simulink model "rtwdemo_shrlib"  (Simulink 7.6)
settings: Solver=FixedStepDiscrete  SolverMode=SingleTasking  StartTime=0.0  StopTime=inf  FixedStep=1  RelTol=1e-3
PostLoadFcn:
  | INC=uint8(1);LIMIT=uint8(4);RESET=uint8(0);K=int32(3);
  | addpath(fullfile((matlabroot), 'toolbox', 'rtw', 'rtwdemos', 'shrlib_demo'));
libraries: rtwdemowidgets x1
Description:
  | Interfacing to Host Simulators Using Shared Libraries
settings Model: Creator=The MathWorks Inc.  ParamWorkspaceSource=ReferencedWorkspace  CovMetricSettings=d  ExtModeTrigMode=oneshot  ExtModeArmWhenConnect=off  ExtModeAutoUpdateStatusClock=off
settings MATStruct: SampleTime=1  Offset=0  Priority=[41.0]
settings DataIOCC: LimitDataPoints=off  SignalLogging=off  SignalLoggingName=sigsOut
settings OptimizationCC: InlineParams=on  InlineInvariantSignals=on  PassReuseOutputArgsAs=Individual arguments  StateBitsets=on  DataBitsets=on  UseTempVars=on  ZeroExternalMemoryAtStartup=off  ZeroInternalMemoryAtStartup=off  NoFixptDivByZeroProtection=on  EfficientFloat2IntCast=on  EfficientMapNaN2IntZero=off  OptimizeModelRefInitCode=on  LifeSpan=1  BufferReusableBoundary=off
settings DebuggingCC: CheckExecutionContextPreStartOutputMsg=on  CheckExecutionContextRuntimeOutputMsg=on  SolverPrmCheckMsg=none  IntegerOverflowMsg=none  StrictBusMsg=ErrorOnBusTreatedAsVector
settings HardwareCC: ProdIntDivRoundTo=Zero  ProdEndianess=LittleEndian  ProdHWDeviceType=Generic->32-bit Embedded Processor  TargetHWDeviceType=Generic->32-bit Embedded Processor
settings ModelReferenceCC: UpdateModelReferenceTargets=IfOutOfDate
settings RTWCC: SystemTargetFile=ert_shrlib.tlc  TLCOptions=-p0 -aWarnNonSaturatedBlocks=0  TemplateMakefile=ert_default_tmf  Description=Real-Time Workshop Embedded Coder (host-based shared library target)  RTWVerbose=off  ProcessScript=ert_shrlib_make_rtw_hook
settings CodeAppCC: ForceParamTrailComments=on  IgnoreCustomStorageClasses=off  IgnoreTestpoints=on
settings STFCustomTargetCC: TargetFcnLib=ansi_tfl_tmw.mat  ParMdlRefBuildCompliant=on  CompOptLevelCompliant=on  CombineOutputUpdateFcns=on  ERTCustomFileBanners=on  SupportNonFinite=off  SupportContinuousTime=off  SupportNonInlinedSFcns=off  ModelStepFunctionPrototypeControlCompliant=on  CPPClassGenCompliant=on  SystemTargetFile=ert_shrlib.tlc
settings ERTTargetCC: TargetFcnLib=ansi_tfl_tmw.mat  MultiwordLength=2048  ERTFirstTimeCompliant=off  SupportNonFinite=off  ExtModeMexFile=noextcomm  InlinedParameterPlacement=NonHierarchical  ERTCustomFileTemplate=example_file_process.tlc  ERTFilePackagingFormat=CompactWithDataFile  ConvertIfToSwitch=off

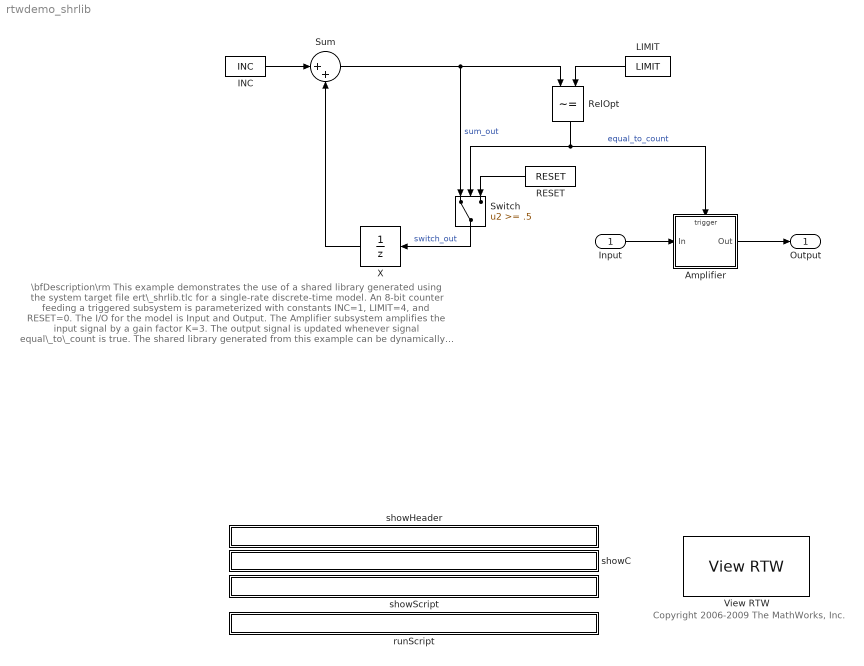
== system rtwdemo_shrlib ==
  note: \bfDescription\rm
      | This example demonstrates the use of a shared library generated using the system target file
      | ert\_shrlib.tlc for a single-rate discrete-time model. An 8-bit counter feeding a triggered
      | subsystem is parameterized with constants INC=1, LIMIT=4, and RESET=0.  The I/O for the model
      | is Input and Output. The Amplifier subsystem amplifies the input signal by a gain factor K=3. The
      | output signal is updated whenever signal equal\_to\_count is true. The shared library generated
      | from this example can be dynamically loaded from another application. See rtwdemo\_shrlib\_app.c
      | for an application example written in C language.
      |
      | \bfInstructions\rm
      | 1. View the Real-Time Workshop configuration by clicking the yellow button below.
      | 2. Double-click the blue button to build and run an example application that uses the generated
      |    shared library. Click the white buttons to view source code.
  note: Copyright 2006-2009 The MathWorks, Inc.
  Input : Inport  OutDataTypeStr=int32  PortDimensions=1  SampleTime=1
  Amplifier : Subsystem  TreatAsAtomicUnit=on
  INC : Constant  Value=INC
  LIMIT : Constant  Value=LIMIT
  RESET : Constant  Value=RESET
  RelOpt : RelationalOperator  Operator=~=  InputSameDT=on
  Sum : Sum  Inputs=|++  InputSameDT=on  OutDataTypeStr=Inherit: Same as first input
  Switch : Switch  Threshold=.5  InputSameDT=on
  View RTW : rtwdemowidgets/View RTW  SystemSampleTime=-1
  X : UnitDelay  SampleTime=-1  StateIdentifier=X
  runScript : Subsystem
      settings: OpenFcn=run_rtwdemo_shrlib_app
      mask Display: disp('Run script run_rtwdemo_shrlib_app.m (double-click)');
  showC : Subsystem
      settings: OpenFcn=edit(fullfile(matlabroot,'toolbox','rtw','rtwdemos', 'shrlib_demo','rtwdemo_shrlib_app.c'))
      mask Display: disp('matlabroot\toolbox\rtw\rtwdemos\shrlib_demo\rtwdemo_shrlib_app.c');
  showHeader : Subsystem
      settings: OpenFcn=edit(fullfile(matlabroot,'toolbox','rtw','rtwdemos', 'shrlib_demo','rtwdemo_shrlib_app.h'))
      mask Display: disp('matlabroot\toolbox\rtw\rtwdemos\shrlib_demo\rtwdemo_shrlib_app.h');
  showScript : Subsystem
      settings: OpenFcn=edit(fullfile(matlabroot,'toolbox','rtw','rtwdemos', 'shrlib_demo','run_rtwdemo_shrlib_app.m'))
      mask Display: disp('matlabroot\toolbox\rtw\rtwdemos\shrlib_demo\run_rtwdemo_shrlib_app.m');
  Output : Outport
  wires:
  INC/1 -> Sum/1
  X/1 -> Sum/2
  Switch/1 -> X/1  "switch_out"
  Sum/1 -> Switch/1, RelOpt/1  "sum_out"
  LIMIT/1 -> RelOpt/2
  Input/1 -> Amplifier/1(In)
  RESET/1 -> Switch/3
  RelOpt/1 -> Switch/2, Amplifier/Trigger  "equal_to_count"
  Amplifier/1(Out) -> Output/1

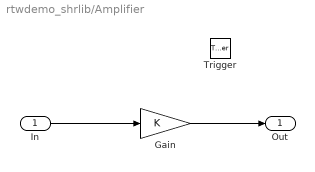
== system rtwdemo_shrlib/Amplifier ==
  In : Inport
  Trigger : TriggerPort
  Gain : Gain  Gain=K  OutDataTypeStr=Inherit: Same as input  ParamDataTypeStr=Inherit: Same as input
  Out : Outport  InitialOutput=0
  wires:
  In/1 -> Gain/1
  Gain/1 -> Out/1

== system rtwdemo_shrlib/runScript ==

== system rtwdemo_shrlib/showC ==

== system rtwdemo_shrlib/showHeader ==

== system rtwdemo_shrlib/showScript ==
